simulink model "twoDimTest"  (R2016b)
settings: Solver=ode4  StartTime=0.0  StopTime=3  FixedStep=0.002  RelTol=1e-3
settings Model: Creator=sskim  LastModifiedBy=sskim

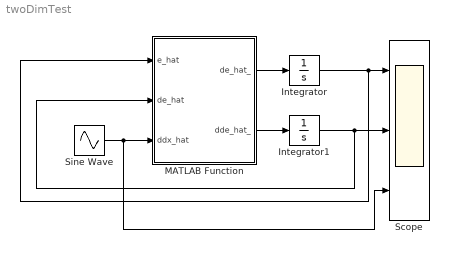
== system twoDimTest ==
  Integrator : Integrator  InitialCondition=0.2
  Integrator1 : Integrator  InitialCondition=0.4
  MATLAB Function : MATLAB Function  TreatAsAtomicUnit=on
  Scope : Scope  NumInputPorts=3
  Sine Wave : Sin  Frequency=0.001  Phase=pi/2  SampleTime=0
  wires:
  Sine Wave/1 -> Scope/3, MATLAB Function/3(ddx_hat)
  MATLAB Function/1(de_hat_) -> Integrator/1
  MATLAB Function/2(dde_hat_) -> Integrator1/1
  Integrator/1 -> MATLAB Function/1(e_hat), Scope/1
  Integrator1/1 -> MATLAB Function/2(de_hat), Scope/2

== matlab function twoDimTest/MATLAB Function ==
  data: e_hat input; de_hat_ output; de_hat input; ddx_hat input; dde_hat_ output
function [de_hat_,dde_hat_] = fcn(e_hat,de_hat,ddx_hat)

de_hat_ = de_hat;
dde_hat_ = -10*e_hat -4*de_hat + ddx_hat;

end
